simulink model "InjCrv_PoI2Cor"  (R2016b)
settings: configuration reference "CodeGenConfigSet" (kept outside this file)
values from neighbouring files (symbols this model uses):
  InjCrv_facPoI2APSQCorEOM_CUR = Calibration.Parameter    [init_InjCrv_PoI2Cor.m]
  InjCrv_facPoI2APSQCorEOM_CURX = Calibration.Parameter    [init_InjCrv_PoI2Cor.m]
  InjCrv_facPoI2APSSOECorEOM_CUR = Calibration.Parameter    [init_InjCrv_PoI2Cor.m]
  InjCrv_facPoI2APSSOECorEOM_CURX = Calibration.Parameter    [init_InjCrv_PoI2Cor.m]
  InjCrv_facPoI2ATSQCorEOM_CUR = Calibration.Parameter    [init_InjCrv_PoI2Cor.m]
  InjCrv_facPoI2ATSQCorEOM_CURX = Calibration.Parameter    [init_InjCrv_PoI2Cor.m]
  InjCrv_facPoI2ATSSOECorEOM_CUR = Calibration.Parameter    [init_InjCrv_PoI2Cor.m]
  InjCrv_facPoI2ATSSOECorEOM_CURX = Calibration.Parameter    [init_InjCrv_PoI2Cor.m]
  InjCrv_facPoI2ETSQCorEOM_CUR = Calibration.Parameter    [init_InjCrv_PoI2Cor.m]
  InjCrv_facPoI2ETSQCorEOM_CURX = Calibration.Parameter    [init_InjCrv_PoI2Cor.m]
  InjCrv_facPoI2ETSSOECorEOM_CUR = Calibration.Parameter    [init_InjCrv_PoI2Cor.m]
  InjCrv_facPoI2ETSSOECorEOM_CURX = Calibration.Parameter    [init_InjCrv_PoI2Cor.m]
  InjCrv_phiPoI2APSCorEOM_MAP = Calibration.Parameter    [init_InjCrv_PoI2Cor.m]
  InjCrv_phiPoI2APSCorEOM_MAPX = Calibration.Parameter    [init_InjCrv_PoI2Cor.m]
  InjCrv_phiPoI2APSCorEOM_MAPY = Calibration.Parameter    [init_InjCrv_PoI2Cor.m]
  InjCrv_phiPoI2ATSCorEOM_MAP = Calibration.Parameter    [init_InjCrv_PoI2Cor.m]
  InjCrv_phiPoI2ATSCorEOM_MAPX = Calibration.Parameter    [init_InjCrv_PoI2Cor.m]
  InjCrv_phiPoI2ATSCorEOM_MAPY = Calibration.Parameter    [init_InjCrv_PoI2Cor.m]
  InjCrv_phiPoI2ETSCorEOM_MAP = Calibration.Parameter    [init_InjCrv_PoI2Cor.m]
  InjCrv_phiPoI2ETSCorEOM_MAPX = Calibration.Parameter    [init_InjCrv_PoI2Cor.m]
  InjCrv_phiPoI2ETSCorEOM_MAPY = Calibration.Parameter    [init_InjCrv_PoI2Cor.m]
  InjCrv_qPoI2APSCorEOM_MAP = Calibration.Parameter    [init_InjCrv_PoI2Cor.m]
  InjCrv_qPoI2APSCorEOM_MAPX = Calibration.Parameter    [init_InjCrv_PoI2Cor.m]
  InjCrv_qPoI2APSCorEOM_MAPY = Calibration.Parameter    [init_InjCrv_PoI2Cor.m]
  InjCrv_qPoI2ATSCorEOM_MAP = Calibration.Parameter    [init_InjCrv_PoI2Cor.m]
  InjCrv_qPoI2ATSCorEOM_MAPX = Calibration.Parameter    [init_InjCrv_PoI2Cor.m]
  InjCrv_qPoI2ATSCorEOM_MAPY = Calibration.Parameter    [init_InjCrv_PoI2Cor.m]
  InjCrv_qPoI2ETSCorEOM_MAP = Calibration.Parameter    [init_InjCrv_PoI2Cor.m]
  InjCrv_qPoI2ETSCorEOM_MAPX = Calibration.Parameter    [init_InjCrv_PoI2Cor.m]
  InjCrv_qPoI2ETSCorEOM_MAPY = Calibration.Parameter    [init_InjCrv_PoI2Cor.m]
  InjCrv_tiPoI2APSCorEOM_MAP = Calibration.Parameter    [init_InjCrv_PoI2Cor.m]
  InjCrv_tiPoI2APSCorEOM_MAPX = Calibration.Parameter    [init_InjCrv_PoI2Cor.m]
  InjCrv_tiPoI2APSCorEOM_MAPY = Calibration.Parameter    [init_InjCrv_PoI2Cor.m]
  InjCrv_tiPoI2ATSCorEOM_MAP = Calibration.Parameter    [init_InjCrv_PoI2Cor.m]
  InjCrv_tiPoI2ATSCorEOM_MAPX = Calibration.Parameter    [init_InjCrv_PoI2Cor.m]
  InjCrv_tiPoI2ATSCorEOM_MAPY = Calibration.Parameter    [init_InjCrv_PoI2Cor.m]
  InjCrv_tiPoI2ETSCorEOM_MAP = Calibration.Parameter    [init_InjCrv_PoI2Cor.m]
  InjCrv_tiPoI2ETSCorEOM_MAPX = Calibration.Parameter    [init_InjCrv_PoI2Cor.m]
  InjCrv_tiPoI2ETSCorEOM_MAPY = Calibration.Parameter    [init_InjCrv_PoI2Cor.m]
settings Model: Creator=Administrator  LastModifiedBy=wangrui
settings ConfigSetRef: SourceLocation=Base Workspace

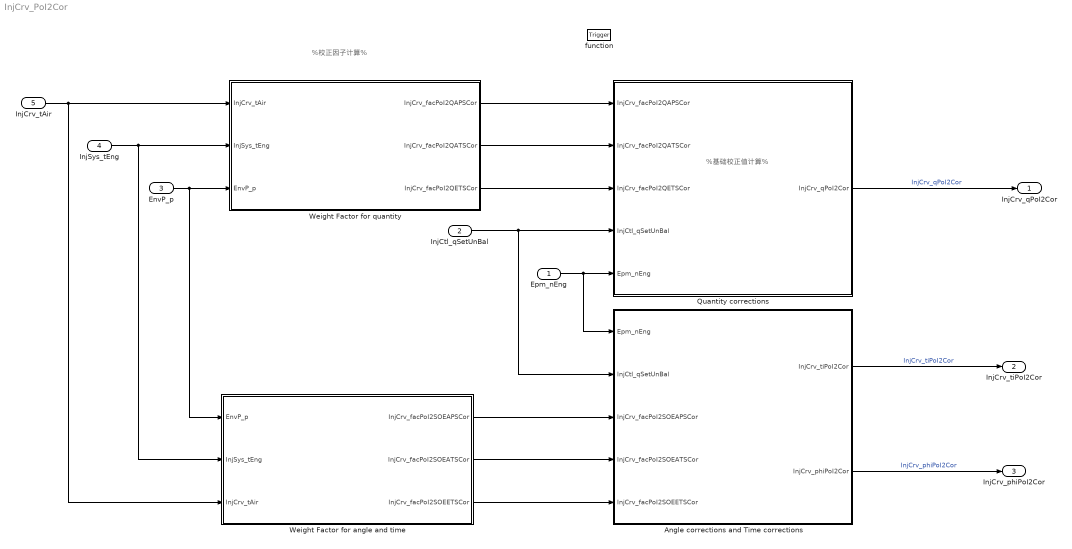
== system InjCrv_PoI2Cor ==
  note: %校正因子计算%
  note: %基础校正值计算%
  Epm_nEng : Inport  Tag=rpm  Description=Engine speed  OutMin=0  OutMax=6000  OutDataTypeStr=EngSpeed_rpm
  InjCtl_qSetUnBal : Inport  Tag=mg/hub  Description=Current injection quantity  Port=2  OutMin=-319  OutMax=319  OutDataTypeStr=FuelMass_mg_hub
  EnvP_p : Inport  Tag=kPa  Description=Barometric pressure  Port=3  OutMin=0  OutMax=3276  OutDataTypeStr=AirPressure_kPa
  InjSys_tEng : Inport  Tag=deg  Description=Engine temperature selected for the injection system  Port=4  OutMin=-1000  OutMax=1000  OutDataTypeStr=Temp_deg
  InjCrv_tAir : Inport  Tag=deg  Description=Air temperature for environment corrections  Port=5  OutMin=-50  OutMax=150  OutDataTypeStr=Temp_deg
  function : TriggerPort  TriggerType=function-call  VariantControl=Variant
  Angle corrections and Time corrections : Subsystem
  Quantity corrections : Subsystem
  Weight Factor for angle and time : Subsystem
  Weight Factor for quantity : Subsystem
  InjCrv_qPoI2Cor : Outport  Tag=mg/hub  Description=PoI2 correction quantity  OutMin=-319  OutMax=319  OutDataTypeStr=FuelMass_mg_hub
  InjCrv_tiPoI2Cor : Outport  Tag=us  Description=PoI2 start of energizing correction time  Port=2  OutMin=-13107  OutMax=13106  OutDataTypeStr=InjTime_us
  InjCrv_phiPoI2Cor : Outport  Tag=CA  Description=PoI2 start of energizing correction angle  Port=3  OutMin=-719  OutMax=719  OutDataTypeStr=Angle_CA
  wires:
  Angle corrections and Time corrections/2(InjCrv_phiPoI2Cor) -> InjCrv_phiPoI2Cor/1  "InjCrv_phiPoI2Cor"
  Angle corrections and Time corrections/1(InjCrv_tiPoI2Cor) -> InjCrv_tiPoI2Cor/1  "InjCrv_tiPoI2Cor"
  Weight Factor for angle and time/3(InjCrv_facPoI2SOEETSCor) -> Angle corrections and Time corrections/5(InjCrv_facPoI2SOEETSCor)
  Weight Factor for angle and time/2(InjCrv_facPoI2SOEATSCor) -> Angle corrections and Time corrections/4(InjCrv_facPoI2SOEATSCor)
  Weight Factor for angle and time/1(InjCrv_facPoI2SOEAPSCor) -> Angle corrections and Time corrections/3(InjCrv_facPoI2SOEAPSCor)
  Weight Factor for quantity/3(InjCrv_facPoI2QETSCor) -> Quantity corrections/3(InjCrv_facPoI2QETSCor)
  Quantity corrections/1(InjCrv_qPoI2Cor) -> InjCrv_qPoI2Cor/1  "InjCrv_qPoI2Cor"
  Weight Factor for quantity/2(InjCrv_facPoI2QATSCor) -> Quantity corrections/2(InjCrv_facPoI2QATSCor)
  Weight Factor for quantity/1(InjCrv_facPoI2QAPSCor) -> Quantity corrections/1(InjCrv_facPoI2QAPSCor)
  InjCtl_qSetUnBal/1 -> Quantity corrections/4(InjCtl_qSetUnBal), Angle corrections and Time corrections/2(InjCtl_qSetUnBal)
  Epm_nEng/1 -> Angle corrections and Time corrections/1(Epm_nEng), Quantity corrections/5(Epm_nEng)
  InjCrv_tAir/1 -> Weight Factor for quantity/1(InjCrv_tAir), Weight Factor for angle and time/3(InjCrv_tAir)
  InjSys_tEng/1 -> Weight Factor for quantity/2(InjSys_tEng), Weight Factor for angle and time/2(InjSys_tEng)
  EnvP_p/1 -> Weight Factor for angle and time/1(EnvP_p), Weight Factor for quantity/3(EnvP_p)

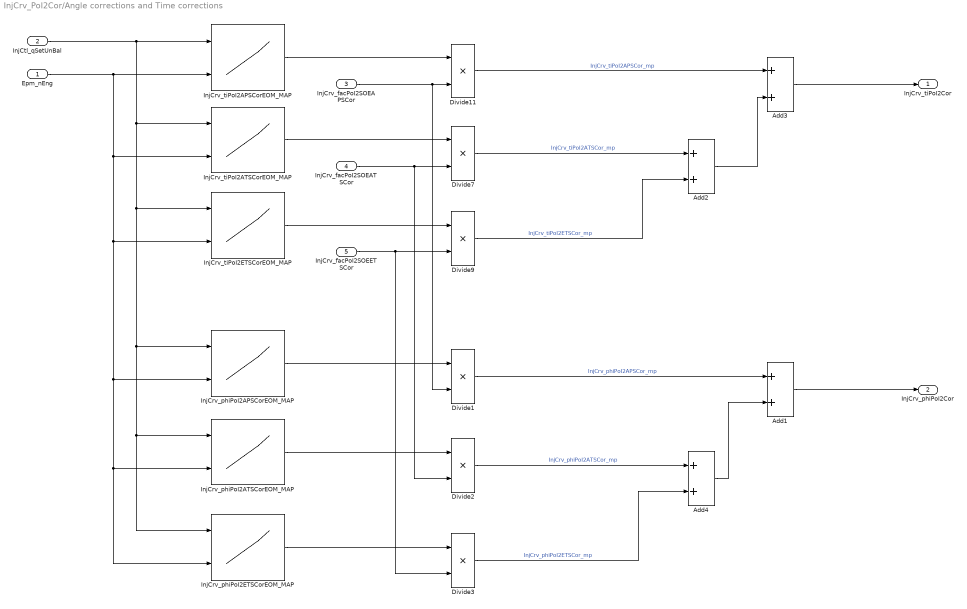
== system InjCrv_PoI2Cor/Angle corrections and Time corrections ==
  Epm_nEng : Inport
  InjCtl_qSetUnBal : Inport  Port=2
  InjCrv_facPoI2SOEAPSCor : Inport  Port=3
  InjCrv_facPoI2SOEATSCor : Inport  Port=4
  InjCrv_facPoI2SOEETSCor : Inport  Port=5
  Add{1..4} (4 alike) : Sum  SaturateOnIntegerOverflow=on  InputSameDT=on
  Divide{1..3,7,9,11} (6 alike) : Product  Inputs=**  OutDataTypeStr=Inherit: Inherit via back propagation  SaturateOnIntegerOverflow=on
  InjCrv_phiPoI2APSCorEOM_MAP : Lookup_n-D  BreakpointsForDimension1=InjCrv_phiPoI2APSCorEOM_MAPY  BreakpointsForDimension2=InjCrv_phiPoI2APSCorEOM_MAPX  IndexSearchMethod=Linear search  BeginIndexSearchUsingPreviousIndexResult=on  Table=InjCrv_phiPoI2APSCorEOM_MAP  ExtrapMethod=Clip  UseLastTableValue=on  InternalRulePriority=Speed  OutDataTypeStr=Inherit: Inherit via back propagation  SaturateOnIntegerOverflow=on
  InjCrv_phiPoI2ATSCorEOM_MAP : Lookup_n-D  BreakpointsForDimension1=InjCrv_phiPoI2ATSCorEOM_MAPY  BreakpointsForDimension2=InjCrv_phiPoI2ATSCorEOM_MAPX  IndexSearchMethod=Linear search  BeginIndexSearchUsingPreviousIndexResult=on  Table=InjCrv_phiPoI2ATSCorEOM_MAP  ExtrapMethod=Clip  UseLastTableValue=on  InternalRulePriority=Speed  OutDataTypeStr=Inherit: Inherit via back propagation  SaturateOnIntegerOverflow=on
  InjCrv_phiPoI2ETSCorEOM_MAP : Lookup_n-D  BreakpointsForDimension1=InjCrv_phiPoI2ETSCorEOM_MAPY  BreakpointsForDimension2=InjCrv_phiPoI2ETSCorEOM_MAPX  IndexSearchMethod=Linear search  BeginIndexSearchUsingPreviousIndexResult=on  Table=InjCrv_phiPoI2ETSCorEOM_MAP  ExtrapMethod=Clip  UseLastTableValue=on  InternalRulePriority=Speed  OutDataTypeStr=Inherit: Inherit via back propagation  SaturateOnIntegerOverflow=on
  InjCrv_tiPoI2APSCorEOM_MAP : Lookup_n-D  BreakpointsForDimension1=InjCrv_tiPoI2APSCorEOM_MAPY  BreakpointsForDimension2=InjCrv_tiPoI2APSCorEOM_MAPX  IndexSearchMethod=Linear search  BeginIndexSearchUsingPreviousIndexResult=on  Table=InjCrv_tiPoI2APSCorEOM_MAP  ExtrapMethod=Clip  UseLastTableValue=on  InternalRulePriority=Speed  OutDataTypeStr=Inherit: Inherit via back propagation  SaturateOnIntegerOverflow=on
  InjCrv_tiPoI2ATSCorEOM_MAP : Lookup_n-D  BreakpointsForDimension1=InjCrv_tiPoI2ATSCorEOM_MAPY  BreakpointsForDimension2=InjCrv_tiPoI2ATSCorEOM_MAPX  IndexSearchMethod=Linear search  BeginIndexSearchUsingPreviousIndexResult=on  Table=InjCrv_tiPoI2ATSCorEOM_MAP  ExtrapMethod=Clip  UseLastTableValue=on  InternalRulePriority=Speed  OutDataTypeStr=Inherit: Inherit via back propagation  SaturateOnIntegerOverflow=on
  InjCrv_tiPoI2ETSCorEOM_MAP : Lookup_n-D  BreakpointsForDimension1=InjCrv_tiPoI2ETSCorEOM_MAPY  BreakpointsForDimension2=InjCrv_tiPoI2ETSCorEOM_MAPX  IndexSearchMethod=Linear search  BeginIndexSearchUsingPreviousIndexResult=on  Table=InjCrv_tiPoI2ETSCorEOM_MAP  ExtrapMethod=Clip  UseLastTableValue=on  InternalRulePriority=Speed  OutDataTypeStr=Inherit: Inherit via back propagation  SaturateOnIntegerOverflow=on
  InjCrv_tiPoI2Cor : Outport
  InjCrv_phiPoI2Cor : Outport  Port=2
  wires:
  Add3/1 -> InjCrv_tiPoI2Cor/1
  Divide9/1 -> Add2/2  "InjCrv_tiPoI2ETSCor_mp"
  InjCrv_facPoI2SOEATSCor/1 -> Divide2/2, Divide7/2
  InjCrv_tiPoI2ETSCorEOM_MAP/1 -> Divide9/1
  Add2/1 -> Add3/2
  Divide7/1 -> Add2/1  "InjCrv_tiPoI2ATSCor_mp"
  InjCrv_facPoI2SOEETSCor/1 -> Divide3/2, Divide9/2
  InjCrv_tiPoI2ATSCorEOM_MAP/1 -> Divide7/1
  Divide11/1 -> Add3/1  "InjCrv_tiPoI2APSCor_mp"
  InjCrv_facPoI2SOEAPSCor/1 -> Divide1/2, Divide11/2
  InjCrv_tiPoI2APSCorEOM_MAP/1 -> Divide11/1
  InjCtl_qSetUnBal/1 -> InjCrv_tiPoI2APSCorEOM_MAP/1, InjCrv_tiPoI2ATSCorEOM_MAP/1, InjCrv_phiPoI2ETSCorEOM_MAP/1, InjCrv_phiPoI2ATSCorEOM_MAP/1, InjCrv_phiPoI2APSCorEOM_MAP/1, InjCrv_tiPoI2ETSCorEOM_MAP/1
  Epm_nEng/1 -> InjCrv_tiPoI2ATSCorEOM_MAP/2, InjCrv_phiPoI2ETSCorEOM_MAP/2, InjCrv_phiPoI2ATSCorEOM_MAP/2, InjCrv_phiPoI2APSCorEOM_MAP/2, InjCrv_tiPoI2ETSCorEOM_MAP/2, InjCrv_tiPoI2APSCorEOM_MAP/2
  InjCrv_phiPoI2APSCorEOM_MAP/1 -> Divide1/1
  InjCrv_phiPoI2ATSCorEOM_MAP/1 -> Divide2/1
  InjCrv_phiPoI2ETSCorEOM_MAP/1 -> Divide3/1
  Divide1/1 -> Add1/1  "InjCrv_phiPoI2APSCor_mp"
  Divide2/1 -> Add4/1  "InjCrv_phiPoI2ATSCor_mp"
  Add4/1 -> Add1/2
  Divide3/1 -> Add4/2  "InjCrv_phiPoI2ETSCor_mp"
  Add1/1 -> InjCrv_phiPoI2Cor/1

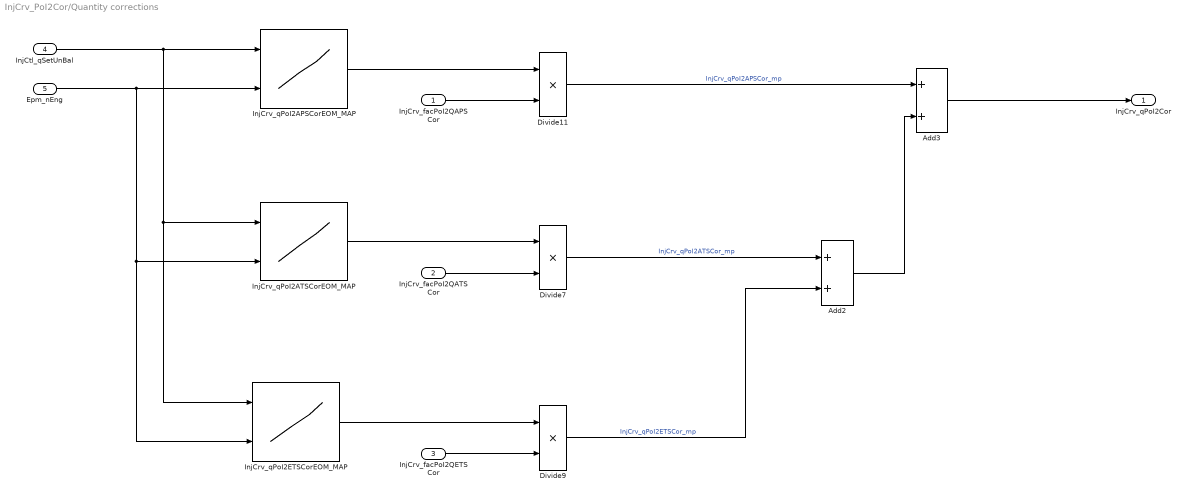
== system InjCrv_PoI2Cor/Quantity corrections ==
  InjCrv_facPoI2QAPSCor : Inport
  InjCrv_facPoI2QATSCor : Inport  Port=2
  InjCrv_facPoI2QETSCor : Inport  Port=3
  InjCtl_qSetUnBal : Inport  Port=4
  Epm_nEng : Inport  Port=5
  Add2 : Sum  SaturateOnIntegerOverflow=on  InputSameDT=on
  Add3 : Sum  SaturateOnIntegerOverflow=on  InputSameDT=on
  Divide11 : Product  Inputs=**  OutDataTypeStr=Inherit: Inherit via back propagation  SaturateOnIntegerOverflow=on
  Divide7 : Product  Inputs=**  OutDataTypeStr=Inherit: Inherit via back propagation  SaturateOnIntegerOverflow=on
  Divide9 : Product  Inputs=**  OutDataTypeStr=Inherit: Inherit via back propagation  SaturateOnIntegerOverflow=on
  InjCrv_qPoI2APSCorEOM_MAP : Lookup_n-D  BreakpointsForDimension1=InjCrv_qPoI2APSCorEOM_MAPY  BreakpointsForDimension2=InjCrv_qPoI2APSCorEOM_MAPX  IndexSearchMethod=Linear search  BeginIndexSearchUsingPreviousIndexResult=on  Table=InjCrv_qPoI2APSCorEOM_MAP  ExtrapMethod=Clip  UseLastTableValue=on  InternalRulePriority=Speed  OutDataTypeStr=Inherit: Inherit via back propagation  SaturateOnIntegerOverflow=on
  InjCrv_qPoI2ATSCorEOM_MAP : Lookup_n-D  BreakpointsForDimension1=InjCrv_qPoI2ATSCorEOM_MAPY  BreakpointsForDimension2=InjCrv_qPoI2ATSCorEOM_MAPX  IndexSearchMethod=Linear search  BeginIndexSearchUsingPreviousIndexResult=on  Table=InjCrv_qPoI2ATSCorEOM_MAP  ExtrapMethod=Clip  UseLastTableValue=on  InternalRulePriority=Speed  OutDataTypeStr=Inherit: Inherit via back propagation  SaturateOnIntegerOverflow=on
  InjCrv_qPoI2ETSCorEOM_MAP : Lookup_n-D  BreakpointsForDimension1=InjCrv_qPoI2ETSCorEOM_MAPY  BreakpointsForDimension2=InjCrv_qPoI2ETSCorEOM_MAPX  IndexSearchMethod=Linear search  BeginIndexSearchUsingPreviousIndexResult=on  Table=InjCrv_qPoI2ETSCorEOM_MAP  ExtrapMethod=Clip  UseLastTableValue=on  InternalRulePriority=Speed  OutDataTypeStr=Inherit: Inherit via back propagation  SaturateOnIntegerOverflow=on
  InjCrv_qPoI2Cor : Outport
  wires:
  Epm_nEng/1 -> InjCrv_qPoI2APSCorEOM_MAP/2, InjCrv_qPoI2ETSCorEOM_MAP/2, InjCrv_qPoI2ATSCorEOM_MAP/2
  InjCtl_qSetUnBal/1 -> InjCrv_qPoI2ETSCorEOM_MAP/1, InjCrv_qPoI2ATSCorEOM_MAP/1, InjCrv_qPoI2APSCorEOM_MAP/1
  InjCrv_qPoI2APSCorEOM_MAP/1 -> Divide11/1
  InjCrv_facPoI2QAPSCor/1 -> Divide11/2
  Divide11/1 -> Add3/1  "InjCrv_qPoI2APSCor_mp"
  InjCrv_qPoI2ATSCorEOM_MAP/1 -> Divide7/1
  InjCrv_facPoI2QETSCor/1 -> Divide9/2
  Divide7/1 -> Add2/1  "InjCrv_qPoI2ATSCor_mp"
  Add2/1 -> Add3/2
  InjCrv_qPoI2ETSCorEOM_MAP/1 -> Divide9/1
  InjCrv_facPoI2QATSCor/1 -> Divide7/2
  Divide9/1 -> Add2/2  "InjCrv_qPoI2ETSCor_mp"
  Add3/1 -> InjCrv_qPoI2Cor/1

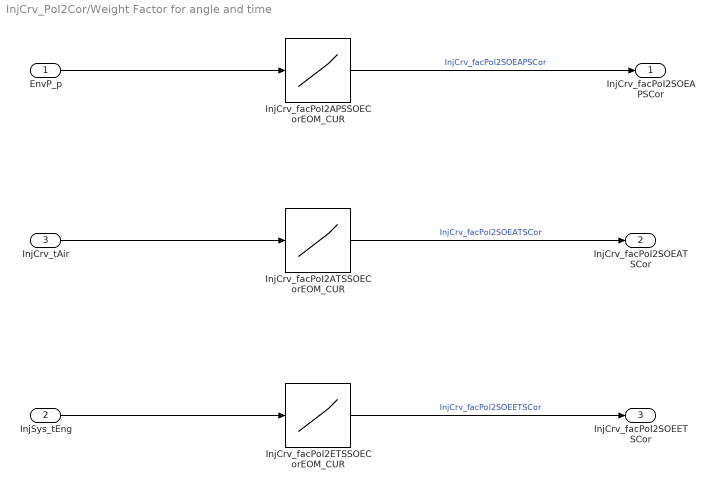
== system InjCrv_PoI2Cor/Weight Factor for angle and time ==
  EnvP_p : Inport
  InjSys_tEng : Inport  Port=2
  InjCrv_tAir : Inport  Port=3
  InjCrv_facPoI2APSSOECorEOM_CUR : Lookup_n-D  NumberOfTableDimensions=1  BreakpointsForDimension1=InjCrv_facPoI2APSSOECorEOM_CURX  IndexSearchMethod=Linear search  BeginIndexSearchUsingPreviousIndexResult=on  Table=InjCrv_facPoI2APSSOECorEOM_CUR  ExtrapMethod=Clip  UseLastTableValue=on  InternalRulePriority=Speed  OutDataTypeStr=Inherit: Inherit via back propagation  SaturateOnIntegerOverflow=on
  InjCrv_facPoI2ATSSOECorEOM_CUR : Lookup_n-D  NumberOfTableDimensions=1  BreakpointsForDimension1=InjCrv_facPoI2ATSSOECorEOM_CURX  IndexSearchMethod=Linear search  BeginIndexSearchUsingPreviousIndexResult=on  Table=InjCrv_facPoI2ATSSOECorEOM_CUR  ExtrapMethod=Clip  UseLastTableValue=on  InternalRulePriority=Speed  OutDataTypeStr=Inherit: Inherit via back propagation  SaturateOnIntegerOverflow=on
  InjCrv_facPoI2ETSSOECorEOM_CUR : Lookup_n-D  NumberOfTableDimensions=1  BreakpointsForDimension1=InjCrv_facPoI2ETSSOECorEOM_CURX  IndexSearchMethod=Linear search  BeginIndexSearchUsingPreviousIndexResult=on  Table=InjCrv_facPoI2ETSSOECorEOM_CUR  ExtrapMethod=Clip  UseLastTableValue=on  InternalRulePriority=Speed  OutDataTypeStr=Inherit: Inherit via back propagation  SaturateOnIntegerOverflow=on
  InjCrv_facPoI2SOEAPSCor : Outport
  InjCrv_facPoI2SOEATSCor : Outport  Port=2
  InjCrv_facPoI2SOEETSCor : Outport  Port=3
  wires:
  EnvP_p/1 -> InjCrv_facPoI2APSSOECorEOM_CUR/1
  InjCrv_facPoI2ETSSOECorEOM_CUR/1 -> InjCrv_facPoI2SOEETSCor/1  "InjCrv_facPoI2SOEETSCor"
  InjCrv_facPoI2ATSSOECorEOM_CUR/1 -> InjCrv_facPoI2SOEATSCor/1  "InjCrv_facPoI2SOEATSCor"
  InjCrv_facPoI2APSSOECorEOM_CUR/1 -> InjCrv_facPoI2SOEAPSCor/1  "InjCrv_facPoI2SOEAPSCor"
  InjCrv_tAir/1 -> InjCrv_facPoI2ATSSOECorEOM_CUR/1
  InjSys_tEng/1 -> InjCrv_facPoI2ETSSOECorEOM_CUR/1

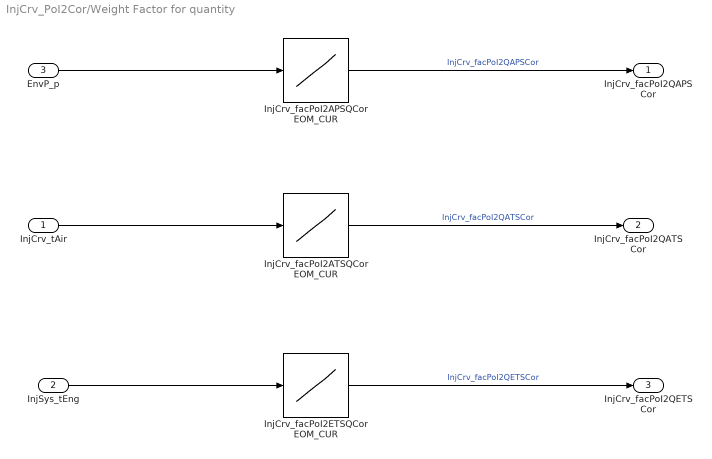
== system InjCrv_PoI2Cor/Weight Factor for quantity ==
  InjCrv_tAir : Inport
  InjSys_tEng : Inport  Port=2
  EnvP_p : Inport  Port=3
  InjCrv_facPoI2APSQCorEOM_CUR : Lookup_n-D  NumberOfTableDimensions=1  BreakpointsForDimension1=InjCrv_facPoI2APSQCorEOM_CURX  IndexSearchMethod=Linear search  BeginIndexSearchUsingPreviousIndexResult=on  Table=InjCrv_facPoI2APSQCorEOM_CUR  ExtrapMethod=Clip  UseLastTableValue=on  InternalRulePriority=Speed  OutDataTypeStr=Inherit: Inherit via back propagation  SaturateOnIntegerOverflow=on
  InjCrv_facPoI2ATSQCorEOM_CUR : Lookup_n-D  NumberOfTableDimensions=1  BreakpointsForDimension1=InjCrv_facPoI2ATSQCorEOM_CURX  IndexSearchMethod=Linear search  BeginIndexSearchUsingPreviousIndexResult=on  Table=InjCrv_facPoI2ATSQCorEOM_CUR  ExtrapMethod=Clip  UseLastTableValue=on  InternalRulePriority=Speed  OutDataTypeStr=Inherit: Inherit via back propagation  SaturateOnIntegerOverflow=on
  InjCrv_facPoI2ETSQCorEOM_CUR : Lookup_n-D  NumberOfTableDimensions=1  BreakpointsForDimension1=InjCrv_facPoI2ETSQCorEOM_CURX  IndexSearchMethod=Linear search  BeginIndexSearchUsingPreviousIndexResult=on  Table=InjCrv_facPoI2ETSQCorEOM_CUR  ExtrapMethod=Clip  UseLastTableValue=on  InternalRulePriority=Speed  OutDataTypeStr=Inherit: Inherit via back propagation  SaturateOnIntegerOverflow=on
  InjCrv_facPoI2QAPSCor : Outport
  InjCrv_facPoI2QATSCor : Outport  Port=2
  InjCrv_facPoI2QETSCor : Outport  Port=3
  wires:
  InjSys_tEng/1 -> InjCrv_facPoI2ETSQCorEOM_CUR/1
  InjCrv_tAir/1 -> InjCrv_facPoI2ATSQCorEOM_CUR/1
  InjCrv_facPoI2APSQCorEOM_CUR/1 -> InjCrv_facPoI2QAPSCor/1  "InjCrv_facPoI2QAPSCor"
  InjCrv_facPoI2ATSQCorEOM_CUR/1 -> InjCrv_facPoI2QATSCor/1  "InjCrv_facPoI2QATSCor"
  InjCrv_facPoI2ETSQCorEOM_CUR/1 -> InjCrv_facPoI2QETSCor/1  "InjCrv_facPoI2QETSCor"
  EnvP_p/1 -> InjCrv_facPoI2APSQCorEOM_CUR/1
